simulink model "Online_Estimation_Synchrongenerator_NEW_2018a"  (R2019a)
settings: Solver=VariableStepAuto  StartTime=0.0  StopTime=20  MaxStep=0.1  MinStep=0.01  RelTol=1e-2  EnableMultiTasking=on
model workspace (MAT data in the model file):
  Ts = 0.001
undefined symbols (not defined in the file or in its folder): gcbh, initializationParams
libraries: ctrlSharedLib x14, simulink x4
settings Model: OrderedModelArguments=off  Creator=The MathWorks, Inc.  LastModifiedBy=Opal3
settings DataIOCC: LimitDataPoints=on  SaveFormat=Array  ReturnWorkspaceOutputs=off
settings OptimizationCC: LifeSpan=inf
settings DebuggingCC: SolverPrmCheckMsg=warning  SFUnexpectedBacktrackingDiag=warning  SFNoUnconditionalDefaultTransitionDiag=warning  SFExecutionAtInitializationDiag=none  ArithmeticOperatorsInVariantConditions=warning
settings HardwareCC: ProdBitPerPointer=32  ProdBitPerSizeT=32  ProdBitPerPtrDiffT=32  ProdLargestAtomicFloat=None  ProdIntDivRoundTo=Undefined  ProdEndianess=Unspecified  ProdWordSize=32  ProdHWDeviceType=32-bit Generic
settings ModelReferenceCC: PropagateSignalLabelsOutOfModel=off
settings SFSimCC: SimUseLocalCustomCode=off  SimGenImportedTypeDefs=on
settings RTWCC: RTWUseLocalCustomCode=off
settings CodeAppCC: StateflowObjectComments=on
settings GRTTargetCC: TargetLangStandard=C89/C90 (ANSI)
settings ConfigComp: CovMetricSettings=dw  CovSaveCumulativeToWorkspaceVar=on  CovSaveSingleToWorkspaceVar=on  CovExternalEMLEnable=off  CovSFcnEnable=off

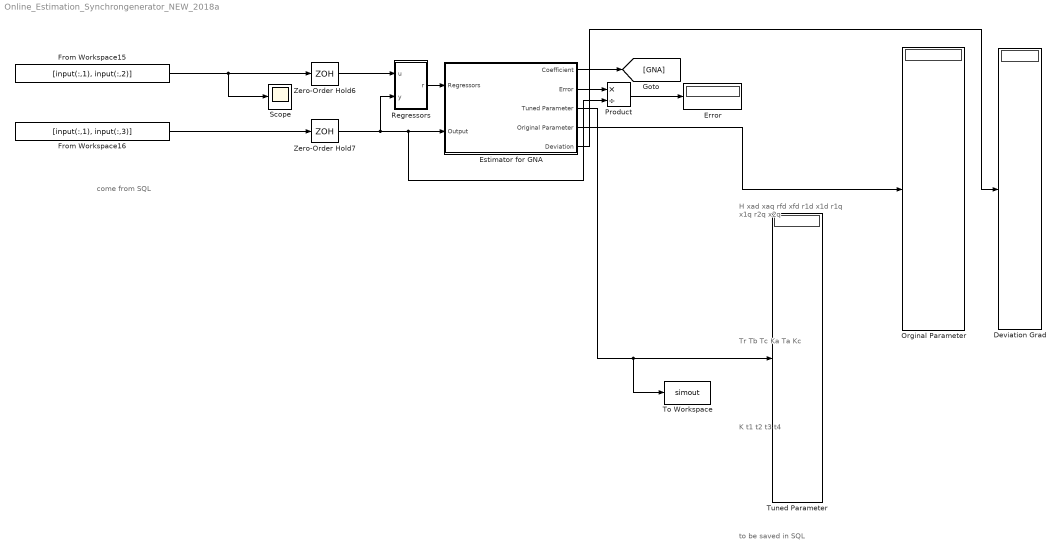
== system Online_Estimation_Synchrongenerator_NEW_2018a ==
  note: to be saved in SQL
  note: K
      | t1
      | t2
      | t3
      | t4
  note: H
      | xad
      | xaq
      | rfd
      | xfd
      | r1d
      | x1d
      | r1q
      | x1q
      | r2q
      | x2q
  note: Tr
      | Tb
      | Tc
      | Ka
      | Ta
      | Kc
  note: come from SQL
  Deviation Grad : Display
  Error : Display
  Estimator for GNA : Subsystem  mask(idEstimatorsRLS){InitialEstimateSource=None, InitialParameterData=12, P0=1, InitialRegressors=0, InitialOutputs=0, History=Infinite, WindowLength=100, EstimationMethod=Normalized Gradient, AdaptationParameter=1-2e-4, HasTimeVaryingAdaptationParameter=off, NormalizationBias=eps, OutputError=on, OutputP=off, AddEnablePort=off, ExternalReset=None, InputProcessing=Sample-based, Ts=Ts}
      mask prompts: InitialEstimateSource "Controllib:blocks:recursiveEstimationMaskInitialEstimate"; InitialParameterData "Controllib:blocks:recursiveEstimationMaskNumberOfParameters"; P0 "Controllib:blocks:recursiveEstimationMaskParameterCovariance"; InitialRegressors "Controllib:blocks:recursiveEstimationMaskInitialRegressors"; InitialOutputs "Controllib:blocks:recursiveEstimationMaskInitialOutputs"; History "Controllib:blocks:recursiveEstimationMaskHistory"; WindowLength "Controllib:blocks:recursiveEstimationMaskWindowLength"; EstimationMethod "AlgorithmForEstimation"; AdaptationParameter "Controllib:blocks:recursiveEstimationMaskAdaptationParameterAG"; HasTimeVaryingAdaptationParameter "Controllib:blocks:recursiveEstimationMaskTimeVarying"; NormalizationBias "Controllib:blocks:recursiveEstimationMaskAdaptationParameterNormalizationBias"; OutputError "Controllib:blocks:recursiveEstimationMaskOutputError"; OutputP "Controllib:blocks:recursiveEstimationMaskOutputCovariance"; AddEnablePort "Controllib:blocks:recursiveEstimationMaskInputEnable"; ExternalReset "Simulink:blkprm_prompts:DelayBlkExternalReset"; InputProcessing "Controllib:blocks:recursiveEstimationMaskInputProcessing"; Ts "Controllib:blocks:recursiveEstimationMaskSampleTime"
      mask help: This online estimation is designed for DT Tuning
      mask init:
      | dlgParams.Ts = Ts;
      | dlgParams.InitialEstimateSource = InitialEstimateSource;
      | dlgParams.InitialParameterData = InitialParameterData;
      | dlgParams.InitialRegressors = InitialRegressors;
      | dlgParams.InitialOutputs = InitialOutputs;
      | dlgParams.P0 = P0;
      | dlgParams.History = History;
      | dlgParams.WindowLength = WindowLength;
      | dlgParams.EstimationMethod = EstimationMethod;
      | dlgParams.AdaptationParameter = AdaptationParameter;
      | dlgParams.NormalizationBias = NormalizationBias;
      | dlgParams.OutputError = OutputError;
      | dlgParams.OutputP = OutputP;
      | dlgParams.AddEnablePort = AddEnablePort;
      | dlgParams.ExternalReset = ExternalReset;
      | dlgParams.InputProcessing = InputProcessing;
      | [initializationParams,algorithmParams,dimParams] = ...
      |     controllib.internal.blocks.rls.maskInitialization(gcbh,dlgParams);
      | % Avoid storing the dlg variables twice in the MaskWSVariables 
      | % block property
      | clear dlgParams;
      mask TypeOptions InitialEstimateSource: Controllib:blocks:recursiveEstimationMaskInitialEstimateNone | Controllib:blocks:recursiveEstimationMaskInitialEstimateInternal | Controllib:blocks:recursiveEstimationMaskInitialEstimateExternal
      mask Callback InitialEstimateSource: controllib.internal.blocks.rls.dialogCallbacks(gcbh,'comboBoxInitialEstimateRLS');
      mask TypeOptions History: Controllib:blocks:recursiveEstimationMaskInfinite | Controllib:blocks:recursiveEstimationMaskFinite
      mask Callback History: controllib.internal.blocks.rls.dialogCallbacks(gcbh,'comboBoxHistory');
      mask TypeOptions EstimationMethod: Controllib:blocks:recursiveEstimationMaskEstimationMethodFF | Controllib:blocks:recursiveEstimationMaskEstimationMethodKF | Controllib:blocks:recursiveEstimationMaskEstimationMethodNG | Controllib:blocks:recursiveEstimationMaskEstimationMethodUG
      mask Callback EstimationMethod: controllib.internal.blocks.rls.dialogCallbacks(gcbh,'comboBoxEstimationMethod');
      mask TypeOptions ExternalReset: delayTheta/ExternalReset | delayL/ExternalReset | delayBuffery/ExternalReset | delayBufferH/ExternalReset | Process Reset/ExternalReset
      mask TypeOptions InputProcessing: Controllib:blocks:recursiveEstimationMaskSampleBased | Controllib:blocks:recursiveEstimationMaskFrameBased
      mask DialogControl EstimatorforOnlineEstimation Prompt: Estimator for Online Estimation
      mask DialogControl containerModelParameters Prompt: GeneratorParameters
      mask DialogControl containerModelStructure Prompt: GeneratorDescription
      mask DialogControl InitialEstimateSource Prompt: Initial Estimate:
      mask DialogControl InitialParameterData Prompt: Number of Parameters:
      mask DialogControl P0 Prompt: Parameter Covariance Matrix:
      mask DialogControl InitialRegressors Prompt: Initial Regressors:
      mask DialogControl InitialOutputs Prompt: Initial Outputs:
      mask DialogControl containerOptions Prompt: Algorithm
      mask DialogControl containerAlgorithmOptions Prompt: Controllib:blocks:recursiveEstimationMaskGroupAlgorithmOpts
      mask DialogControl History Prompt: History:
      mask DialogControl WindowLength Prompt: Window Length:
      mask DialogControl AdaptationParameter Prompt: Adaptation Gain:
      mask DialogControl HasTimeVaryingAdaptationParameter Prompt: Time-varying
      mask DialogControl NormalizationBias Prompt: Normalization Bias:
      mask DialogControl containerBlockOptions Prompt: Controllib:blocks:recursiveEstimationMaskGroupBlockOpts
      mask DialogControl OutputError Prompt: Output estimation error
      mask DialogControl OutputP Prompt: Output parameter covariance matrix
      mask DialogControl AddEnablePort Prompt: Add enable port
      mask DialogControl ExternalReset Prompt: External reset:
      mask DialogControl InputProcessing Prompt: Input Processing:
      mask DialogControl Ts Prompt: Sample Time (-1 for inherited):
  From Workspace15 : FromWorkspace  VariableName=[input(:,1), input(:,2)]
  From Workspace16 : FromWorkspace  VariableName=[input(:,1), input(:,3)]
  Orginal Parameter : Display
  Product : Product  Inputs=*/
  Regressors : Subsystem
  Scope : Scope
  To Workspace : ToWorkspace  VariableName=simout  SaveFormat=Timeseries  SampleTime=-1
  Tuned Parameter : Display
  Zero-Order Hold6 : ZeroOrderHold  SampleTime=Ts
  Zero-Order Hold7 : ZeroOrderHold  SampleTime=Ts
  wires:
  From Workspace16/1 -> Zero-Order Hold7/1
  From Workspace15/1 -> Scope/1, Zero-Order Hold6/1
  Zero-Order Hold6/1 -> Regressors/1(u)
  Product/1 -> Error/1
  Zero-Order Hold7/1 -> Estimator for GNA/2(Output), Product/2, Regressors/2(y)
  Regressors/1(r) -> Estimator for GNA/1(Regressors)
  Estimator for GNA/1(Coefficient) -> [GNA]
  Estimator for GNA/2(Error) -> Product/1
  Estimator for GNA/4(Original Parameter) -> Orginal Parameter/1
  Estimator for GNA/5(Deviation) -> Deviation Grad/1
  Estimator for GNA/3(Tuned Parameter) -> To Workspace/1, Tuned Parameter/1

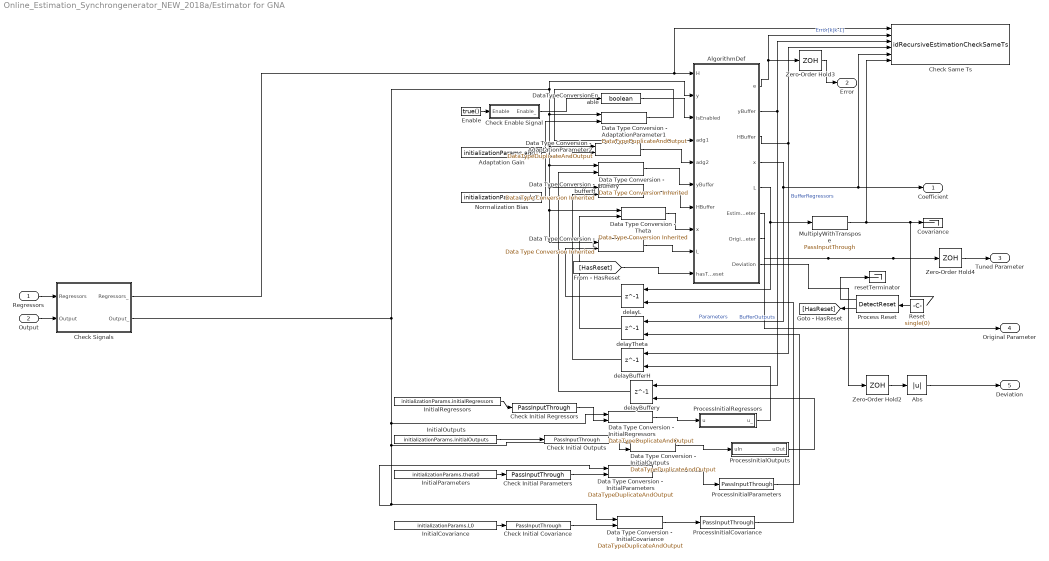
== system Online_Estimation_Synchrongenerator_NEW_2018a/Estimator for GNA ==
  Regressors : Inport
  Output : Inport  Port=2
  Abs : Abs
  Adaptation Gain : Constant  Value=initializationParams.adg1  OutDataTypeStr=Inherit: Inherit via back propagation
  AlgorithmDef : MATLAB Function  TreatAsAtomicUnit=on  SystemSampleTime=Ts
  Check Enable Signal : Subsystem
  Check Initial Covariance : ctrlSharedLib/Utilities/PassInputThrough  SystemSampleTime=-1
      settings: SourceProductName=Control System Toolbox  SourceProductBaseCode=CT
  Check Initial Outputs : ctrlSharedLib/Utilities/PassInputThrough  SystemSampleTime=-1
      settings: SourceProductName=Control System Toolbox  SourceProductBaseCode=CT
  Check Initial Parameters : ctrlSharedLib/Utilities/PassInputThrough  SystemSampleTime=-1
      settings: SourceProductName=Control System Toolbox  SourceProductBaseCode=CT
  Check Initial Regressors : ctrlSharedLib/Utilities/PassInputThrough  SystemSampleTime=-1
      settings: SourceProductName=Control System Toolbox  SourceProductBaseCode=CT
  Check Same Ts : S-Function  FunctionName=idRecursiveEstimationCheckSameTs  Parameters=get_param(gcbh,'Parent'), uint16(6)  SFunctionDeploymentMode=off  EnableBusSupport=off
  Check Signals : Subsystem
      mask init:
      | csp = controllib.internal.blocks.rls.maskInitializationCheckSignals(gcbh);
  Covariance : Terminator
  Data Type Conversion - AdaptationParameter1 : ctrlSharedLib/Utilities/DataTypeDuplicateAndOutput  SystemSampleTime=-1
      settings: SourceProductName=Control System Toolbox  SourceProductBaseCode=CT
  Data Type Conversion - AdaptationParameter2 : ctrlSharedLib/Utilities/DataTypeDuplicateAndOutput  SystemSampleTime=-1
      settings: SourceProductName=Control System Toolbox  SourceProductBaseCode=CT
  Data Type Conversion - InitialCovariance : ctrlSharedLib/Utilities/DataTypeDuplicateAndOutput  SystemSampleTime=-1
      settings: SourceProductName=Control System Toolbox  SourceProductBaseCode=CT
  Data Type Conversion - InitialOutputs : ctrlSharedLib/Utilities/DataTypeDuplicateAndOutput  SystemSampleTime=-1
      settings: SourceProductName=Control System Toolbox  SourceProductBaseCode=CT
  Data Type Conversion - InitialParameters : ctrlSharedLib/Utilities/DataTypeDuplicateAndOutput  SystemSampleTime=-1
      settings: SourceProductName=Control System Toolbox  SourceProductBaseCode=CT
  Data Type Conversion - InitialRegressors : ctrlSharedLib/Utilities/DataTypeDuplicateAndOutput  SystemSampleTime=-1
      settings: SourceProductName=Control System Toolbox  SourceProductBaseCode=CT
  Data Type Conversion - L : simulink/Signal Attributes/Data Type Conversion Inherited  ConvertRealWorld=Real World Value  DoSatur=off
      settings: SourceProductName=Simulink  SourceProductBaseCode=SL
  Data Type Conversion - Theta : simulink/Signal Attributes/Data Type Conversion Inherited  ConvertRealWorld=Real World Value  DoSatur=off
      settings: SourceProductName=Simulink  SourceProductBaseCode=SL
  Data Type Conversion - bufferH : simulink/Signal Attributes/Data Type Conversion Inherited  ConvertRealWorld=Real World Value  DoSatur=off
      settings: SourceProductName=Simulink  SourceProductBaseCode=SL
  Data Type Conversion - buffery : simulink/Signal Attributes/Data Type Conversion Inherited  ConvertRealWorld=Real World Value  DoSatur=off
      settings: SourceProductName=Simulink  SourceProductBaseCode=SL
  DataTypeConversionEnable : DataTypeConversion  OutDataTypeStr=boolean
  Enable : Constant  Value=true()  OutDataTypeStr=boolean
  InitialCovariance : Constant  Value=initializationParams.L0  OutDataTypeStr=Inherit: Inherit via back propagation
  InitialOutputs : Constant  Value=initializationParams.initialOutputs  VectorParams1D=off  OutDataTypeStr=Inherit: Inherit via back propagation
  InitialParameters : Constant  Value=initializationParams.theta0  VectorParams1D=off  OutDataTypeStr=Inherit: Inherit via back propagation
  InitialRegressors : Constant  Value=initializationParams.initialRegressors  VectorParams1D=off  OutDataTypeStr=Inherit: Inherit via back propagation
  MultiplyWithTranspose : ctrlSharedLib/Utilities/PassInputThrough  SystemSampleTime=-1
      settings: SourceProductName=Control System Toolbox  SourceProductBaseCode=CT
  Normalization Bias : Constant  Value=initializationParams.adg2  OutDataTypeStr=Inherit: Inherit via back propagation
  Process Reset : ctrlSharedLib/Utilities/DetectReset
      settings: SourceProductName=Control System Toolbox  SourceProductBaseCode=CT
  ProcessInitialCovariance : ctrlSharedLib/Utilities/PassInputThrough  SystemSampleTime=-1
      settings: SourceProductName=Control System Toolbox  SourceProductBaseCode=CT
  ProcessInitialOutputs : Subsystem  mask(idRProcessInitialOutputs){}
  ProcessInitialParameters : ctrlSharedLib/Utilities/PassInputThrough  SystemSampleTime=-1
      settings: SourceProductName=Control System Toolbox  SourceProductBaseCode=CT
  ProcessInitialRegressors : Subsystem  mask(rlsProcessInitialRegressors){}
  Reset : Constant  Value=single(0)
  Zero-Order Hold2 : ZeroOrderHold  SampleTime=5
  Zero-Order Hold3 : ZeroOrderHold  SampleTime=5
  Zero-Order Hold4 : ZeroOrderHold  SampleTime=0.5
  delayBufferH : Delay  DelayLength=1  InitialConditionSource=Input port
      settings: InputPortMap=u0,p4
  delayBuffery : Delay  DelayLength=1  InitialConditionSource=Input port
      settings: InputPortMap=u0,p4
  delayL : Delay  DelayLength=1  InitialConditionSource=Input port
      settings: InputPortMap=u0,p4
  delayTheta : Delay  DelayLength=1  InitialConditionSource=Input port
      settings: InputPortMap=u0,p4
  resetTerminator : Terminator
  Coefficient : Outport
  Error : Outport  Port=2  VectorParamsAs1DForOutWhenUnconnected=on
  Tuned Parameter : Outport  Port=3  VectorParamsAs1DForOutWhenUnconnected=on
  Original Parameter : Outport  Port=4  VectorParamsAs1DForOutWhenUnconnected=on
  Deviation : Outport  Port=5  VectorParamsAs1DForOutWhenUnconnected=on
  wires:
  Process Reset/1 -> resetTerminator/1
  [HasReset] -> AlgorithmDef/10(hasTriggeredReset)
  Process Reset/2 -> [HasReset]
  ProcessInitialRegressors/1(u_) -> delayBufferH/2
  ProcessInitialOutputs/1(uOut) -> delayBuffery/2
  Data Type Conversion - InitialOutputs/1 -> ProcessInitialOutputs/1(uIn)
  Data Type Conversion - InitialRegressors/1 -> ProcessInitialRegressors/1(u)
  Check Initial Regressors/1 -> Data Type Conversion - InitialRegressors/2
  InitialOutputs/1 -> Check Initial Outputs/1
  InitialRegressors/1 -> Check Initial Regressors/1
  Check Initial Outputs/1 -> Data Type Conversion - InitialOutputs/2
  ProcessInitialParameters/1 -> delayTheta/2
  ProcessInitialCovariance/1 -> delayL/2
  delayBufferH/1 -> Data Type Conversion - bufferH/2
  delayBuffery/1 -> Data Type Conversion - buffery/2
  Data Type Conversion - buffery/1 -> AlgorithmDef/6("yBuffer ")
  Data Type Conversion - bufferH/1 -> AlgorithmDef/7("HBuffer ")
  AlgorithmDef/2(yBuffer) -> delayBuffery/1, Check Same Ts/3  "BufferOutputs"
  AlgorithmDef/3(HBuffer) -> delayBufferH/1, Check Same Ts/4  "BufferRegressors"
  Check Initial Covariance/1 -> Data Type Conversion - InitialCovariance/2
  Check Initial Parameters/1 -> Data Type Conversion - InitialParameters/2
  Data Type Conversion - Theta/1 -> AlgorithmDef/8("x ")
  AlgorithmDef/4(x) -> delayTheta/1, Check Same Ts/5, Coefficient/1  "Parameters"
  Normalization Bias/1 -> Data Type Conversion - AdaptationParameter2/2
  Data Type Conversion - AdaptationParameter2/1 -> AlgorithmDef/5(adg2)
  MultiplyWithTranspose/1 -> Covariance/1, Check Same Ts/6
  Check Signals/2(Output_) -> AlgorithmDef/2(y), Data Type Conversion - L/1, Data Type Conversion - Theta/1, Data Type Conversion - bufferH/1, Data Type Conversion - buffery/1, Data Type Conversion - AdaptationParameter2/1, Data Type Conversion - AdaptationParameter1/1, Data Type Conversion - InitialRegressors/1, Data Type Conversion - InitialOutputs/1, Data Type Conversion - InitialParameters/1, Data Type Conversion - InitialCovariance/1
  Check Signals/1(Regressors_) -> Check Same Ts/1, AlgorithmDef/1(H)
  Check Enable Signal/1(Enable_) -> DataTypeConversionEnable/1
  Regressors/1 -> Check Signals/1(Regressors)
  Output/1 -> Check Signals/2(Output)
  InitialParameters/1 -> Check Initial Parameters/1
  InitialCovariance/1 -> Check Initial Covariance/1
  Data Type Conversion - InitialCovariance/1 -> ProcessInitialCovariance/1
  Data Type Conversion - InitialParameters/1 -> ProcessInitialParameters/1
  Enable/1 -> Check Enable Signal/1(Enable)
  DataTypeConversionEnable/1 -> AlgorithmDef/3(isEnabled)
  Reset/1 -> Process Reset/1
  delayL/1 -> Data Type Conversion - L/2
  Adaptation Gain/1 -> Data Type Conversion - AdaptationParameter1/2
  Data Type Conversion - L/1 -> AlgorithmDef/9("L ")
  delayTheta/1 -> Data Type Conversion - Theta/2
  AlgorithmDef/1(e) -> Check Same Ts/2, Zero-Order Hold3/1  "Error[k|k-1]"
  Data Type Conversion - AdaptationParameter1/1 -> AlgorithmDef/4(adg1)
  AlgorithmDef/5(L) -> delayL/1, MultiplyWithTranspose/1
  AlgorithmDef/7(OriginalParameter) -> Original Parameter/1
  AlgorithmDef/8(Deviation) -> Zero-Order Hold2/1
  Abs/1 -> Deviation/1
  Zero-Order Hold2/1 -> Abs/1
  Zero-Order Hold3/1 -> Error/1
  AlgorithmDef/6(EstimatedParameter) -> Zero-Order Hold4/1
  Zero-Order Hold4/1 -> Tuned Parameter/1

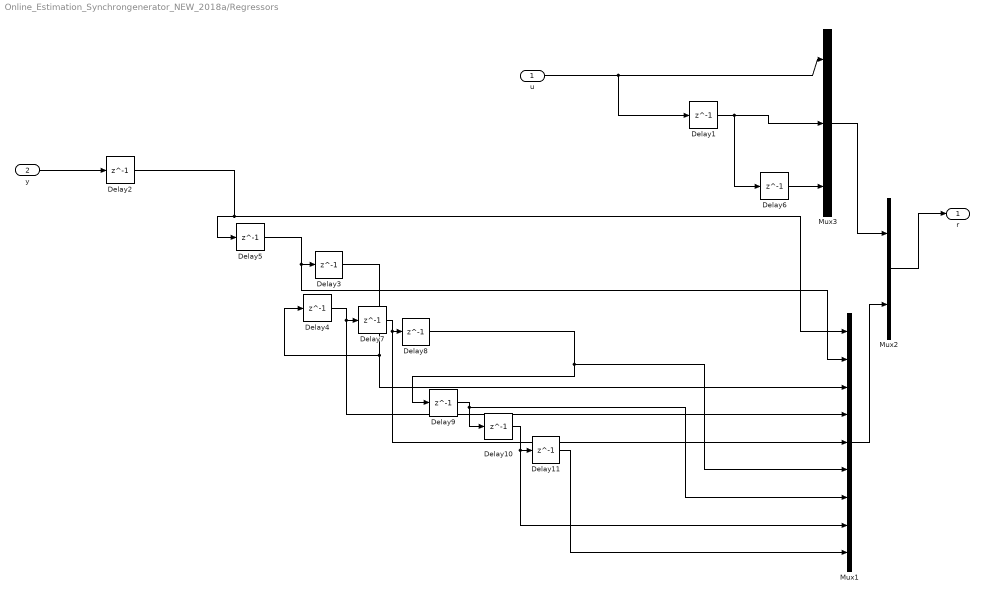
== system Online_Estimation_Synchrongenerator_NEW_2018a/Regressors ==
  u : Inport
  y : Inport  Port=2
  Delay1 : Delay  DelayLength=1  InitialCondition=1  SampleTime=Ts
  Delay{2..5,7..11} (9 alike) : Delay  DelayLength=1  InitialCondition=2  SampleTime=Ts
  Delay6 : Delay  DelayLength=1  InitialCondition=1  SampleTime=Ts
  Mux1 : Mux  Inputs=9
  Mux2 : Mux  Inputs=2
  Mux3 : Mux  Inputs=3
  r : Outport
  wires:
  Mux2/1 -> r/1
  Delay1/1 -> Delay6/1, Mux3/2
  y/1 -> Delay2/1
  Mux3/1 -> Mux2/1
  u/1 -> Delay1/1, Mux3/1
  Delay2/1 -> Delay5/1, Mux1/1
  Delay5/1 -> Delay3/1, Mux1/2
  Mux1/1 -> Mux2/2
  Delay3/1 -> Delay4/1, Mux1/3
  Delay4/1 -> Delay7/1, Mux1/4
  Delay6/1 -> Mux3/3
  Delay7/1 -> Delay8/1, Mux1/5
  Delay8/1 -> Delay9/1, Mux1/6
  Delay9/1 -> Delay10/1, Mux1/7
  Delay10/1 -> Delay11/1, Mux1/8
  Delay11/1 -> Mux1/9

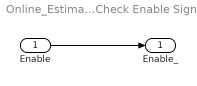
== system Online_Estimation_Synchrongenerator_NEW_2018a/Estimator for GNA/Check Enable Signal ==
  Enable : Inport
  Enable_ : Outport
  wires:
  Enable/1 -> Enable_/1

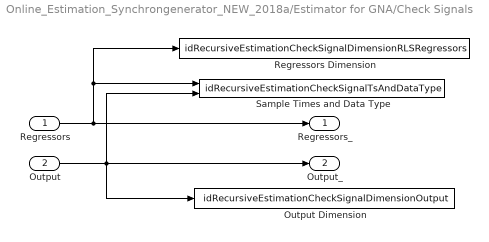
== system Online_Estimation_Synchrongenerator_NEW_2018a/Estimator for GNA/Check Signals ==
  Regressors : Inport
  Output : Inport  Port=2
  Output Dimension : S-Function  FunctionName=idRecursiveEstimationCheckSignalDimensionOutput  Parameters=csp.estimatorBlockPath, csp.isUsingFrames  SFunctionDeploymentMode=off  EnableBusSupport=off
  Regressors Dimension : S-Function  FunctionName=idRecursiveEstimationCheckSignalDimensionRLSRegressors  Parameters=csp.estimatorBlockPath, csp.isInitialEstimateSourceInternal, algorithmParams.nParameters, csp.isUsingFrames  SFunctionDeploymentMode=off  EnableBusSupport=off
  Sample Times and Data Type : S-Function  FunctionName=idRecursiveEstimationCheckSignalTsAndDataType  Parameters=csp.estimatorBlockPath, Ts, 'Regressors', 'Output',algorithmParams.nParameters  SFunctionDeploymentMode=off  EnableBusSupport=off
  Regressors_ : Outport
  Output_ : Outport  Port=2
  wires:
  Regressors/1 -> Regressors_/1, Sample Times and Data Type/1, Regressors Dimension/1
  Output/1 -> Sample Times and Data Type/2, Output Dimension/1, Output_/1

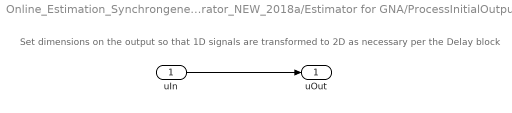
== system Online_Estimation_Synchrongenerator_NEW_2018a/Estimator for GNA/ProcessInitialOutputs ==
  note: Set dimensions on the output so that 1D signals are transformed to 2D as necessary per the Delay block
  uIn : Inport
  uOut : Outport  PortDimensions=dimParams.Outputs.yBuffer
  wires:
  uIn/1 -> uOut/1

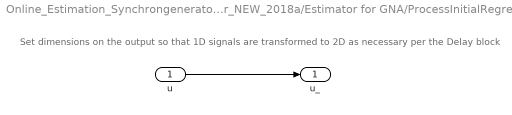
== system Online_Estimation_Synchrongenerator_NEW_2018a/Estimator for GNA/ProcessInitialRegressors ==
  note: Set dimensions on the output so that 1D signals are transformed to 2D as necessary per the Delay block
  u : Inport
  u_ : Outport  PortDimensions=dimParams.Outputs.HBuffer
  wires:
  u/1 -> u_/1

== matlab function Online_Estimation_Synchrongenerator_NEW_2018a/Estimator for GNA/AlgorithmDef ==
  settings: updateMethod=DISCRETE  sampleTime=Ts
  data: e output; H input; yBuffer output size=algorithmParams.nParameters; HBuffer output; x output; L output; y input; isEnabled input size=1; adg1 input; adg2 input; yBuffer input size=dimParams.Outputs.yBuffer; HBuffer input size=dimParams.Outputs.HBuffer; x input size=dimParams.Outputs.x; L input size=dimParams.Outputs.L; hasTriggeredReset input size=1; algorithmParams parameter; EstimatedParameter output; OriginalParameter output; Deviation output
function [e,yBuffer,HBuffer,x,L,EstimatedParameter,OriginalParameter,Deviation] = Parameterestimation(...
    H,y,... 
    isEnabled,adg1,adg2,... 
    yBuffer,HBuffer,x,L,... 
    hasTriggeredReset,...   
    algorithmParams)






persistent rlsEstimator;
if isempty(rlsEstimator)
    rlsEstimator = controllib.internal.blocks.rls.getEstimator(algorithmParams);
end


if hasTriggeredReset
    [x,L] = rlsEstimator.reset(yBuffer,HBuffer,x,L);
end

% Estimate 
[yBuffer,HBuffer,x,L,e] = rlsEstimator.estimate(...
    yBuffer, HBuffer, x, L,... % states
    y, H,... % new IO data
    isEnabled, adg1, adg2, algorithmParams); % helper variables

OriginalParameterGenerator=[6.705882,0.0018,0.055704,0.019,0.0076,0.17,0.18,0.00087]; % Original Parameter= [H,rfd, rld, rlq, r2q, xddd, xqdd, rstr ]
OriginalParameterExicter=[0.01,0.05,0.05,100,0.01,0.1]; % Tr, Tb, Tc, Ka, Ta, Kc
OriginalParameterTurbine=[5,0.5,0.1,0.95,0.8]; % K, t1, t2, t3, t4
% Max und Minimum

Tolerance=1e-5;
[Synparameter,ExParameter,Tuparameter]=rlsEstimation_Gen(x,Tolerance,OriginalParameterGenerator,OriginalParameterExicter,OriginalParameterTurbine);

Deviation_G=(Synparameter-OriginalParameterGenerator)./OriginalParameterGenerator;
Deviation_E=(ExParameter-OriginalParameterExicter)./OriginalParameterExicter;
Deviation_T=(Tuparameter-OriginalParameterTurbine)./OriginalParameterTurbine;

OriginalParameter=[OriginalParameterGenerator,OriginalParameterExicter,OriginalParameterTurbine];
EstimatedParameter=[Synparameter,ExParameter,Tuparameter];
Deviation=[Deviation_G,Deviation_E,Deviation_T];
end
